simulink model "ASW_DcycGen"  (R2023a)
settings: configuration reference "cfg_FastTaskCodeGeneration_v01" (kept outside this file)
undefined symbols (not defined in the file): Cdbl_tiFstTaskSmpTi
settings Model: DataDictionary=dd_foc_dictionary.sldd  EnableAccessToBaseWorkspace=off  Creator=WFYXQ  LastModifiedBy=xiaoqiang.yuan
settings ConfigSetRef: SourceName=cfg_FastTaskCodeGeneration_v01

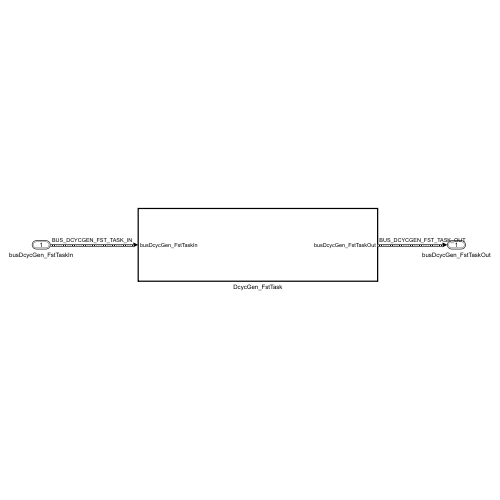
[thumbnail: Simulink's stored preview of the top-level diagram]
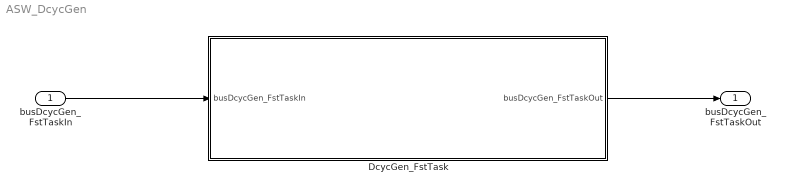
== system ASW_DcycGen ==
  busDcycGen_FstTaskIn : Inport  OutDataTypeStr=Bus: BUS_DCYCGEN_FST_TASK_IN  SampleTime=round(double(Cdbl_tiFstTaskSmpTi),8)  BusOutputAsStruct=on
  DcycGen_FstTask : Subsystem  TreatAsAtomicUnit=on  RTWFcnName=DcycGen_FstTask
      settings: RTWSystemCode=Nonreusable function  RTWFcnNameOpts=User specified
  busDcycGen_FstTaskOut : Outport  OutDataTypeStr=Bus: BUS_DCYCGEN_FST_TASK_OUT  SampleTime=round(double(Cdbl_tiFstTaskSmpTi),8)
  wires:
  busDcycGen_FstTaskIn/1 -> DcycGen_FstTask/1(busDcycGen_FstTaskIn)
  DcycGen_FstTask/1(busDcycGen_FstTaskOut) -> busDcycGen_FstTaskOut/1

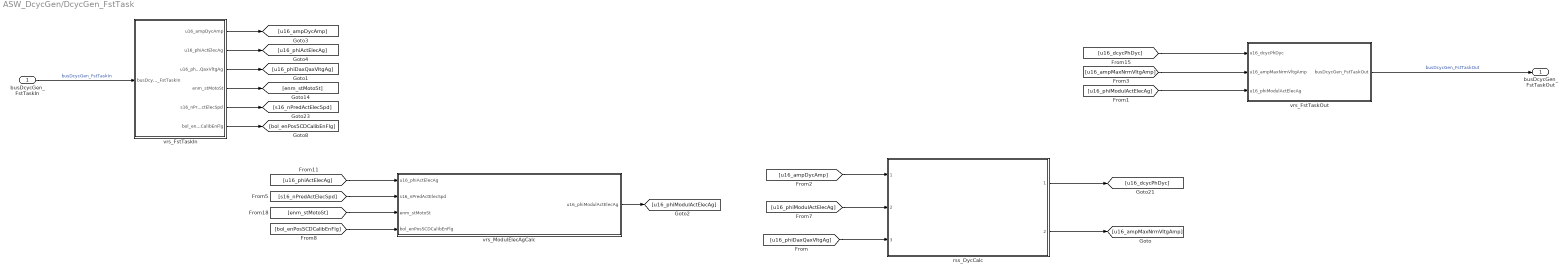
== system ASW_DcycGen/DcycGen_FstTask ==
  busDcycGen_FstTaskIn : Inport
  rss_DycCalc : Subsystem  ReferencedSubsystem=rss_DycCalc
  vrs_FstTaskIn : Subsystem  Variant=on  VariantControlMode=label  VariantControl=Choice  LabelModeActiveChoice=cstSensCtrlLbl
  vrs_FstTaskOut : Subsystem  Variant=on  VariantControlMode=label  VariantControl=Choice  LabelModeActiveChoice=cstSensCtrlLbl
  vrs_ModulElecAgCalc : Subsystem  Variant=on  VariantControlMode=label  VariantControl=Choice  LabelModeActiveChoice=cstSensCtrlLbl
  busDcycGen_FstTaskOut : Outport
  wires:
  [u16_phiModulActElecAg] -> vrs_FstTaskOut/3(u16_phiModulActElecAg)
  [u16_ampMaxNrmVltgAmp] -> vrs_FstTaskOut/2(u16_ampMaxNrmVltgAmp)
  vrs_FstTaskIn/4(enm_stMotoSt) -> [enm_stMotoSt]
  vrs_FstTaskIn/1(u16_ampDycAmp) -> [u16_ampDycAmp]
  vrs_FstTaskOut/1(busDcycGen_FstTaskOut) -> busDcycGen_FstTaskOut/1  "busDcycGen_FstTaskOut"
  [u16_phiDaxQaxVltgAg] -> rss_DycCalc/3
  vrs_FstTaskIn/5(s16_nPredActElecSpd) -> [s16_nPredActElecSpd]
  rss_DycCalc/1 -> [u16_dcycPhDyc]
  vrs_FstTaskIn/2(u16_phiActElecAg) -> [u16_phiActElecAg]
  busDcycGen_FstTaskIn/1 -> vrs_FstTaskIn/1(busDcycGen_FstTaskIn)  "busDcycGen_FstTaskIn"
  [u16_dcycPhDyc] -> vrs_FstTaskOut/1(u16_dcycPhDyc)
  [u16_ampDycAmp] -> rss_DycCalc/1
  rss_DycCalc/2 -> [u16_ampMaxNrmVltgAmp]
  [u16_phiModulActElecAg] -> rss_DycCalc/2
  vrs_FstTaskIn/3(u16_phiDaxQaxVltgAg) -> [u16_phiDaxQaxVltgAg]
  vrs_FstTaskIn/6(bol_enPosSCDCalibEnFlg) -> [bol_enPosSCDCalibEnFlg]
  [u16_phiActElecAg] -> vrs_ModulElecAgCalc/1(u16_phiActElecAg)
  [s16_nPredActElecSpd] -> vrs_ModulElecAgCalc/2(s16_nPredActElecSpd)
  [enm_stMotoSt] -> vrs_ModulElecAgCalc/3(enm_stMotoSt)
  [bol_enPosSCDCalibEnFlg] -> vrs_ModulElecAgCalc/4(bol_enPosSCDCalibEnFlg)
  vrs_ModulElecAgCalc/1(u16_phiModulActElecAg) -> [u16_phiModulActElecAg]

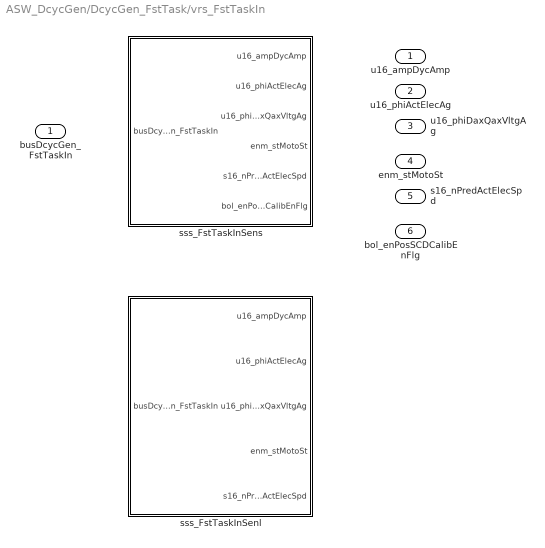
== system ASW_DcycGen/DcycGen_FstTask/vrs_FstTaskIn ==
  busDcycGen_FstTaskIn : Inport
  sss_FstTaskInSenl : Subsystem  VariantControl=cstSenlCtrlLbl
  sss_FstTaskInSens : Subsystem  VariantControl=cstSensCtrlLbl
  u16_ampDycAmp : Outport
  u16_phiActElecAg : Outport  Port=2
  u16_phiDaxQaxVltgAg : Outport  Port=3
  enm_stMotoSt : Outport  Port=4
  s16_nPredActElecSpd : Outport  Port=5
  bol_enPosSCDCalibEnFlg : Outport  Port=6

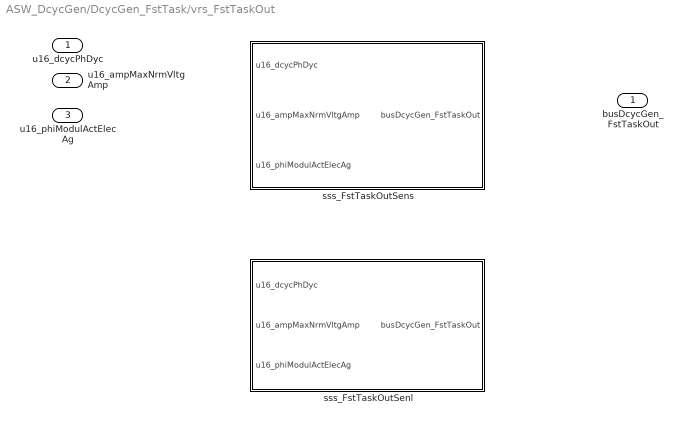
== system ASW_DcycGen/DcycGen_FstTask/vrs_FstTaskOut ==
  u16_dcycPhDyc : Inport
  u16_ampMaxNrmVltgAmp : Inport  Port=2
  u16_phiModulActElecAg : Inport  Port=3
  sss_FstTaskOutSenl : Subsystem  VariantControl=cstSenlCtrlLbl
  sss_FstTaskOutSens : Subsystem  VariantControl=cstSensCtrlLbl
  busDcycGen_FstTaskOut : Outport

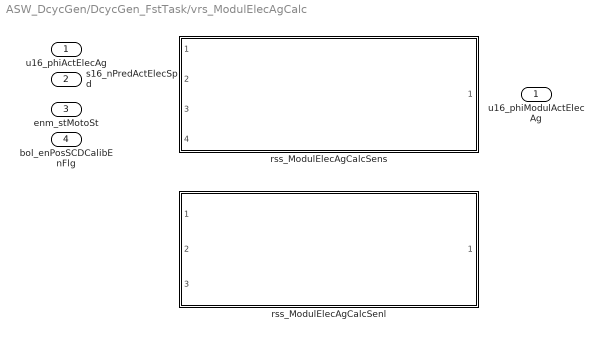
== system ASW_DcycGen/DcycGen_FstTask/vrs_ModulElecAgCalc ==
  u16_phiActElecAg : Inport
  s16_nPredActElecSpd : Inport  Port=2
  enm_stMotoSt : Inport  Port=3
  bol_enPosSCDCalibEnFlg : Inport  Port=4
  rss_ModulElecAgCalcSenl : Subsystem  VariantControl=cstSenlCtrlLbl  ReferencedSubsystem=rss_ModulElecAgCalcSenl
  rss_ModulElecAgCalcSens : Subsystem  VariantControl=cstSensCtrlLbl  ReferencedSubsystem=rss_ModulElecAgCalcSens
  u16_phiModulActElecAg : Outport

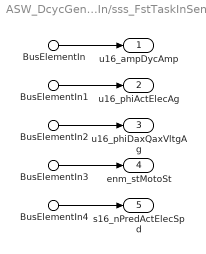
== system ASW_DcycGen/DcycGen_FstTask/vrs_FstTaskIn/sss_FstTaskInSenl ==
  BusElementIn : Inport  PortName=busDcycGen_FstTaskIn  Element=u16_ampDycAmp
  BusElementIn1 : Inport  PortName=busDcycGen_FstTaskIn  Element=u16_phiActElecAg
  BusElementIn2 : Inport  PortName=busDcycGen_FstTaskIn  Element=u16_phiDaxQaxVltgAg
  BusElementIn3 : Inport  PortName=busDcycGen_FstTaskIn  Element=enm_stMotoSt
  BusElementIn4 : Inport  PortName=busDcycGen_FstTaskIn  Element=s16_nPredActElecSpd
  u16_ampDycAmp : Outport
  u16_phiActElecAg : Outport  Port=2
  u16_phiDaxQaxVltgAg : Outport  Port=3
  enm_stMotoSt : Outport  Port=4
  s16_nPredActElecSpd : Outport  Port=5
  wires:
  BusElementIn/1 -> u16_ampDycAmp/1
  BusElementIn1/1 -> u16_phiActElecAg/1
  BusElementIn2/1 -> u16_phiDaxQaxVltgAg/1
  BusElementIn3/1 -> enm_stMotoSt/1
  BusElementIn4/1 -> s16_nPredActElecSpd/1

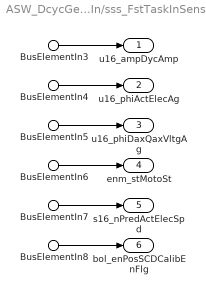
== system ASW_DcycGen/DcycGen_FstTask/vrs_FstTaskIn/sss_FstTaskInSens ==
  BusElementIn3 : Inport  PortName=busDcycGen_FstTaskIn  Element=u16_ampDycAmp
  BusElementIn4 : Inport  PortName=busDcycGen_FstTaskIn  Element=u16_phiActElecAg
  BusElementIn5 : Inport  PortName=busDcycGen_FstTaskIn  Element=u16_phiDaxQaxVltgAg
  BusElementIn6 : Inport  PortName=busDcycGen_FstTaskIn  Element=enm_stMotoSt
  BusElementIn7 : Inport  PortName=busDcycGen_FstTaskIn  Element=s16_nPredActElecSpd
  BusElementIn8 : Inport  PortName=busDcycGen_FstTaskIn  Element=bol_enPosSCDCalibEnFlg
  u16_ampDycAmp : Outport
  u16_phiActElecAg : Outport  Port=2
  u16_phiDaxQaxVltgAg : Outport  Port=3
  enm_stMotoSt : Outport  Port=4
  s16_nPredActElecSpd : Outport  Port=5
  bol_enPosSCDCalibEnFlg : Outport  Port=6
  wires:
  BusElementIn3/1 -> u16_ampDycAmp/1
  BusElementIn4/1 -> u16_phiActElecAg/1
  BusElementIn5/1 -> u16_phiDaxQaxVltgAg/1
  BusElementIn6/1 -> enm_stMotoSt/1
  BusElementIn7/1 -> s16_nPredActElecSpd/1
  BusElementIn8/1 -> bol_enPosSCDCalibEnFlg/1

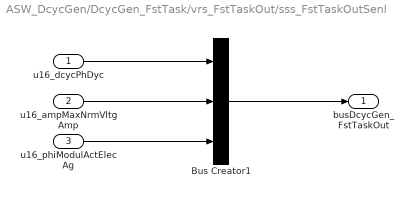
== system ASW_DcycGen/DcycGen_FstTask/vrs_FstTaskOut/sss_FstTaskOutSenl ==
  u16_dcycPhDyc : Inport
  u16_ampMaxNrmVltgAmp : Inport  Port=2
  u16_phiModulActElecAg : Inport  Port=3
  Bus Creator1 : BusCreator  Inputs=3  OutDataTypeStr=Bus: BUS_DCYCGEN_FST_TASK_OUT  NonVirtualBus=on
      settings: InheritFromInputs=off
  busDcycGen_FstTaskOut : Outport
  wires:
  u16_dcycPhDyc/1 -> Bus Creator1/1
  u16_ampMaxNrmVltgAmp/1 -> Bus Creator1/2
  u16_phiModulActElecAg/1 -> Bus Creator1/3
  Bus Creator1/1 -> busDcycGen_FstTaskOut/1

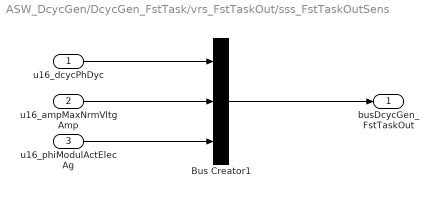
== system ASW_DcycGen/DcycGen_FstTask/vrs_FstTaskOut/sss_FstTaskOutSens ==
  u16_dcycPhDyc : Inport
  u16_ampMaxNrmVltgAmp : Inport  Port=2
  u16_phiModulActElecAg : Inport  Port=3
  Bus Creator1 : BusCreator  Inputs=3  OutDataTypeStr=Bus: BUS_DCYCGEN_FST_TASK_OUT  NonVirtualBus=on
      settings: InheritFromInputs=off
  busDcycGen_FstTaskOut : Outport
  wires:
  u16_dcycPhDyc/1 -> Bus Creator1/1
  u16_ampMaxNrmVltgAmp/1 -> Bus Creator1/2
  u16_phiModulActElecAg/1 -> Bus Creator1/3
  Bus Creator1/1 -> busDcycGen_FstTaskOut/1
